simulink library "carnotUIBK"  (R2018b)
settings: Solver=VariableStepAuto  StartTime=0.0  StopTime=10.0  RelTol=1e-3  EnableMultiTasking=on
values from neighbouring files (symbols this model uses):
  A = 7*10*2    (= 140)    [theta_ground_v1.m]    (also in xlswrite1.m = num2cell(data))
  amb_factor = 1    [DOOR.m]    (also in WALL.m; WINDOW.m = 0)
  area = obj.width * obj.height    [DOOR.m]    (also in RES.m = []; ROOM.m = 0; THERMALZONE.m = area + room(kk).area; WALL.m = area - obj.doors(jj).calc_area())
  B = A/(0.5 * P)    (= 8.23529411765)    [theta_ground_v1.m]
  boundary = BOUNDARY()    [BUILDING.m]    (also in WALL.m = '')
  building = obj    [BUILDING.m]    (also in create_building_automatic.m = building.save(); ini_building_automatic.m = building.add_variant_hvac(building.variant_hvac, hvac); load_building_automatic.m = building.save())
  C = zeros(1,length(d)+1)    [CONSTRUCTION.m]    (also in DOOR.m = [0 0 0]; WALL.m = [0 0 0]; WINDOW.m = [0 0 0])
  control = 2    [GAIN.m]    (also in GAINS.m)
  cp = str2num(value)    [CONSTRUCTION.m]
  height = 0    [DOOR.m]    (also in ROOM.m; THERMALZONE.m; WALL.m; WINDOW.m)
  p = [timevec_weather weather(:,12)]    [BOUNDARY.m]    (also in WEATHER.m = 0; init_carnotUIBK.m = cell2mat(carnotUIBKpaths(i,2)))
  rho = str2num(value)    [CONSTRUCTION.m]    (also in theta_ground_v1.m = 2000)
  type = 1    [CONSTRUCTION.m]    (also in GAINS.m = raw_moisture{ii,3}; STRUCTURE.m = 0)
  view_factor = 1    [DOOR.m]    (also in WINDOW.m = 0)
  wall = []    [ROOM.m]
  z = obj.Z    [WALL.m]    (also in theta_ground_v1.m = 0)
  zone = obj.zone(ind)    [THERMALZONE.m]
undefined symbols (not defined in the file or in its folder): const, Dd, get_building, pos, Qdot_C, Qdot_H, Qdot_I_electricity, Qdot_I_light, Qdot_I_person, Qdot_S, Qdot_T_ground, Qdot_T_neighbour, Qdot_T_opaque, Qdot_T_window, Qdot_V_infiltration, Qdot_V_mech, Qdot_V_window, r_frame, solar_ratio, solar_ratio1, solar_ratio2, Tc, Tr, Ts, Uvalue, wallsurface, window, window_height, window_heigth, window_width, windowsurface, x_CO2, x_H2O, x_VOC
libraries: carnot x104, simulink x16, $bdroot x16, simulink_extras x14
(part 2 of 12)

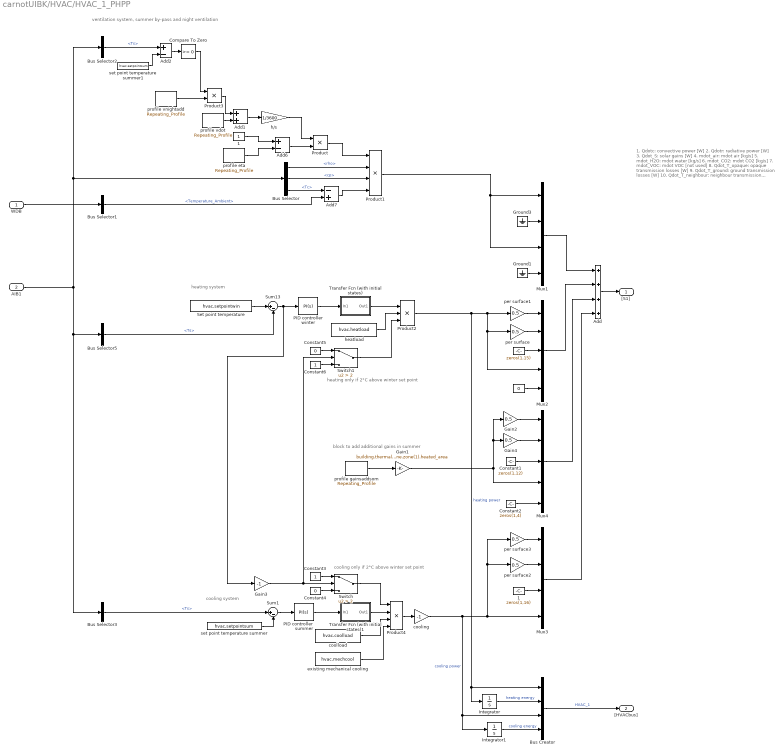
== system carnotUIBK/HVAC/HVAC_1_PHPP ==
  note: cooling only if 2°C above winter set point
  note: block to add additional gains in summer
  note: heating only if 2°C above winter set point
  note: 1.	Qdotc: convective power [W]
      | 2.	Qdotr: radiative power [W]
      | 3.	Qdot_S: solar gains [W]
      | 4.	mdot_air: mdot air [kg/s]
      | 5.	mdot_H2O: mdot water [kg/s]
      | 6.	mdot_CO2: mdot CO2 [kg/s]
      | 7.	mdot_VOC: mdot VOC [not used]
      | 8.	Qdot_T_opaque: opaque transmission losses [W]
      | 9.	Qdot_T_ground: ground transmission losses [W]
      | 10.	Qdot_T_neighbour: neighbour transmission losses [W]
      | 11.	Qdot_T_window: window transmission losses [W]
      | 12.	Qdot_V_mech: mechanical ventilation losses [W]
      | 13.	Qdot_V_window: window ventilation losses [W]
      | 14.	Qdot_V_infiltration: infiltration ventilation losses [W]
      | 15.	Qdot_I_person: person internal gains [W]
      | 16.	Qdot_I_light: light internal gains [W]
      | 17.	Qdot_I_electricity: electricity internal gains [W]
      | 18.	Qdot_H: heating power [W]
      | 19.	Qdot_C: cooling power [W]
  note: heating system
  note: cooling system
  note: ventilation system, summer by-pass and night ventilation
  WDB : Inport
  AIB1 : Inport  Port=2
  " " : Constant  Value=0
  "   " : Constant  Value=zeros(1,15)
  "   1" : Constant  Value=zeros(1,16)
  1 : Constant
  Add : Sum  Inputs=++++
  Add1 : Sum
  Add2 : Sum  Inputs=+-
  Add6 : Sum  Inputs=+-
  Add7 : Sum  Inputs=-+
  Bus Creator : BusCreator  Inputs=4
  Bus Selector : BusSelector  OutputSignals=rho,cp,Tc
  Bus Selector1 : BusSelector  OutputSignals=Temperature_Ambient
  Bus Selector2 : BusSelector  OutputSignals=Ts
  Bus Selector3 : BusSelector  OutputSignals=Ts
  Bus Selector5 : BusSelector  OutputSignals=Ts
  Compare To Zero : simulink/Logic and Bit Operations/Compare To Zero  relop=>=  OutDataTypeStr=boolean
  Constant1 : Constant  Value=zeros(1,12)
  Constant2 : Constant  Value=zeros(1,4)
  Constant3 : Constant
  Constant4 : Constant  Value=0
  Constant5 : Constant  Value=0
  Constant6 : Constant
  Gain1 : Gain  Gain=building.thermalzone.zone(1).heated_area  SaturateOnIntegerOverflow=on  OutDataTypeStr=Inherit: Same as input  ParamDataTypeStr=Inherit: Same as input
  Gain2 : Gain  Gain=0.5  SaturateOnIntegerOverflow=on  OutDataTypeStr=Inherit: Same as input  ParamDataTypeStr=Inherit: Same as input
  Gain3 : Gain  Gain=-1  SaturateOnIntegerOverflow=on  OutDataTypeStr=Inherit: Same as input  ParamDataTypeStr=Inherit: Same as input
  Gain4 : Gain  Gain=0.5  SaturateOnIntegerOverflow=on  OutDataTypeStr=Inherit: Same as input  ParamDataTypeStr=Inherit: Same as input
  Ground1 : Ground
  Ground3 : Ground
  Integrator : Integrator
  Integrator1 : Integrator
  Mux1 : Mux  Inputs=[1 10 1 7]
  Mux2 : Mux  Inputs=[1 1 15 1 1]
  Mux3 : Mux  Inputs=[1 1 16 1]
  Mux4 : Mux  Inputs=[1 1 12 1 4]
  PID controller summer : simulink/Continuous/PID Controller  Controller=PI  Form=Ideal  TimeDomain=Continuous-time  SampleTime=-1  IntegratorMethod=Forward Euler  FilterMethod=Forward Euler  ControllerParametersSource=internal  P=hvac.valves.Kp  I=(1/(hvac.valves.Tn*60))  D=0  UseFilter=on  N=100  TunerSelectOption=Transfer Function Based (PID Tuner App)  InitialConditionSource=internal  InitialConditionForIntegrator=0  InitialConditionForFilter=0  DifferentiatorICPrevScaledInput=0  ExternalReset=none  TrackingMode=off  Kt=1  LimitOutput=on  UpperSaturationLimit=hvac.valves.valve_up  LowerSaturationLimit=hvac.valves.valve_low  LinearizeAsGain=off  AntiWindupMode=clamping  Kb=1  POutMin=[]  POutMax=[]  IOutMin=[]  IOutMax=[]  DOutMin=[]  DOutMax=[]  NOutMin=[]  NOutMax=[]  SumOutMin=[]  SumOutMax=[]  SaturationOutMin=[]  SaturationOutMax=[]  PParamMin=[]  PParamMax=[]  IParamMin=[]  IParamMax=[]  DParamMin=[]  DParamMax=[]  NParamMin=[]  NParamMax=[]  KbParamMin=[]  KbParamMax=[]  KtParamMin=[]  KtParamMax=[]  KbOutMin=[]  KbOutMax=[]  KtOutMin=[]  KtOutMax=[]  IntegratorOutMin=[]  IntegratorOutMax=[]  FilterOutMin=[]  FilterOutMax=[]  SumI1OutMin=[]  SumI1OutMax=[]  SumI2OutMin=[]  SumI2OutMax=[]  SumI3OutMin=[]  SumI3OutMax=[]  SumI4OutMin=[]  SumI4OutMax=[]  SumDOutMin=[]  SumDOutMax=[]  DifferentiatorOutMin=[]  DifferentiatorOutMax=[]  FilterDiffOutCoefMin=[]  FilterDiffOutCoefMax=[]  ReciprocalOutMin=[]  ReciprocalOutMax=[]  SumDenOutMin=[]  SumDenOutMax=[]  SumNumOutMin=[]  SumNumOutMax=[]  DivideOutMin=[]  DivideOutMax=[]  IntegratorContinuousStateAttributes=''  IntegratorStateMustResolveToSignalObject=off  IntegratorRTWStateStorageClass=Auto  FilterContinuousStateAttributes=''  FilterStateMustResolveToSignalObject=off  FilterRTWStateStorageClass=Auto  ParallelPVariant=Passthrough  IdealPVariant=InternalParameters  IVariant=InternalParameters  DVariant=Disabled  IntegratorVariant=Continuous  SatVariant=Enabled  AWVariant=ContClampingIdeal  PCopyVariant=InternalParamsIdeal  TRVariant=Disabled  FdbkBlocksVariant=Forward  IdealPFdbkVariant=Disabled  SatFdbkVariant=Disabled  DerivativeFilterVariant=Disabled  NVariant=Disabled  NCopyVariant=Disabled_SignalSpec  FilterICVariant=Disabled  IntegratorICVariant=InternalICs  ExternalResetVariant=Disabled  TRSumVariant=Passthrough  SumFdbkVariant=Disabled  SumVariant=Sum_PI
  PID controller winter : simulink/Continuous/PID Controller  Controller=PI  Form=Ideal  TimeDomain=Continuous-time  SampleTime=-1  IntegratorMethod=Forward Euler  FilterMethod=Forward Euler  ControllerParametersSource=internal  P=hvac.valves.Kp  I=(1/(hvac.valves.Tn*60))  D=0  UseFilter=on  N=100  TunerSelectOption=Transfer Function Based (PID Tuner App)  InitialConditionSource=internal  InitialConditionForIntegrator=0  InitialConditionForFilter=0  DifferentiatorICPrevScaledInput=0  ExternalReset=none  TrackingMode=off  Kt=1  LimitOutput=on  UpperSaturationLimit=hvac.valves.valve_up  LowerSaturationLimit=hvac.valves.valve_low  LinearizeAsGain=off  AntiWindupMode=clamping  Kb=1  POutMin=[]  POutMax=[]  IOutMin=[]  IOutMax=[]  DOutMin=[]  DOutMax=[]  NOutMin=[]  NOutMax=[]  SumOutMin=[]  SumOutMax=[]  SaturationOutMin=[]  SaturationOutMax=[]  PParamMin=[]  PParamMax=[]  IParamMin=[]  IParamMax=[]  DParamMin=[]  DParamMax=[]  NParamMin=[]  NParamMax=[]  KbParamMin=[]  KbParamMax=[]  KtParamMin=[]  KtParamMax=[]  KbOutMin=[]  KbOutMax=[]  KtOutMin=[]  KtOutMax=[]  IntegratorOutMin=[]  IntegratorOutMax=[]  FilterOutMin=[]  FilterOutMax=[]  SumI1OutMin=[]  SumI1OutMax=[]  SumI2OutMin=[]  SumI2OutMax=[]  SumI3OutMin=[]  SumI3OutMax=[]  SumI4OutMin=[]  SumI4OutMax=[]  SumDOutMin=[]  SumDOutMax=[]  DifferentiatorOutMin=[]  DifferentiatorOutMax=[]  FilterDiffOutCoefMin=[]  FilterDiffOutCoefMax=[]  ReciprocalOutMin=[]  ReciprocalOutMax=[]  SumDenOutMin=[]  SumDenOutMax=[]  SumNumOutMin=[]  SumNumOutMax=[]  DivideOutMin=[]  DivideOutMax=[]  IntegratorContinuousStateAttributes=''  IntegratorStateMustResolveToSignalObject=off  IntegratorRTWStateStorageClass=Auto  FilterContinuousStateAttributes=''  FilterStateMustResolveToSignalObject=off  FilterRTWStateStorageClass=Auto  ParallelPVariant=Passthrough  IdealPVariant=InternalParameters  IVariant=InternalParameters  DVariant=Disabled  IntegratorVariant=Continuous  SatVariant=Enabled  AWVariant=ContClampingIdeal  PCopyVariant=InternalParamsIdeal  TRVariant=Disabled  FdbkBlocksVariant=Forward  IdealPFdbkVariant=Disabled  SatFdbkVariant=Disabled  DerivativeFilterVariant=Disabled  NVariant=Disabled  NCopyVariant=Disabled_SignalSpec  FilterICVariant=Disabled  IntegratorICVariant=InternalICs  ExternalResetVariant=Disabled  TRSumVariant=Passthrough  SumFdbkVariant=Disabled  SumVariant=Sum_PI
  Product : Product
  Product1 : Product  Inputs=4
  Product2 : Product  Inputs=3
  Product3 : Product
  Product4 : Product  Inputs=4
  Set point temperature : Constant  Value=hvac.setpointwin  VectorParams1D=off
  Sum1 : Sum  Inputs=|+-
  Sum13 : Sum  Inputs=|+-
  Switch : Switch  Criteria=u2 > Threshold  Threshold=2
  Switch1 : Switch  Criteria=u2 > Threshold  Threshold=2
  Transfer Fcn (with initial states) : Subsystem  mask(Transfer Function with Initial States){N=[1], D=[300  1], X0=0}
      mask prompts: N "Numerator:"; D "Denominator:"; X0 "Initial conditions:"
      mask help: Vector expressions for numerator, and denominator. Coefficients are in descending powers of s.
      mask init:
      | [A,B,C,Dd]=tf2ss(N,D);if (isempty(X0));[m,n]=size(A);X0=zeros(1,m); end;
      mask Help: Specify the initial states for the transfer function.  The state ordering is determined by the m-file tf2ss.  There is no unique mapping of the states in a transfer function to states in a state-space representation.  However, tf2ss will consistently use the same mapping for a given transfer function.
      mask Display: dpoly(N,D,'s')
  Transfer Fcn (with initial states)1 : Subsystem  mask(Transfer Function with Initial States){N=[1], D=[300  1], X0=0}
      mask prompts: N "Numerator:"; D "Denominator:"; X0 "Initial conditions:"
      mask help: Vector expressions for numerator, and denominator. Coefficients are in descending powers of s.
      mask init:
      | [A,B,C,Dd]=tf2ss(N,D);if (isempty(X0));[m,n]=size(A);X0=zeros(1,m); end;
      mask Help: Specify the initial states for the transfer function.  The state ordering is determined by the m-file tf2ss.  There is no unique mapping of the states in a transfer function to states in a state-space representation.  However, tf2ss will consistently use the same mapping for a given transfer function.
      mask Display: dpoly(N,D,'s')
  cooling : Gain  Gain=-1  SaturateOnIntegerOverflow=on  OutDataTypeStr=Inherit: Same as input  ParamDataTypeStr=Inherit: Same as input
  coolload : Constant  Value=hvac.coolload
  existing mechanical cooling : Constant  Value=hvac.mechcool
  h/s : Gain  Gain=1/3600
  heatload : Constant  Value=hvac.heatload
  per surface{,1..3} (4 alike) : Gain  Gain=0.5  SaturateOnIntegerOverflow=on  OutDataTypeStr=Inherit: Same as input  ParamDataTypeStr=Inherit: Same as input
  profile eta : carnot/Load/General/Repeating_Profile  period=hvac.eta.time(end)  rep_seq_t=hvac.eta.time(1:end-1)  rep_seq_d=hvac.eta.duration  rep_seq_y=hvac.eta.value
  profile gainsaddsom : carnot/Load/General/Repeating_Profile  period=hvac.gainsum.time(end)  rep_seq_t=hvac.gainsum.time(1:end-1)  rep_seq_d=hvac.gainsum.duration  rep_seq_y=hvac.gainsum.value
  profile vdot : carnot/Load/General/Repeating_Profile  period=hvac.vdot_winsom.time(end)  rep_seq_t=hvac.vdot_winsom.time(1:end-1)  rep_seq_d=hvac.vdot_winsom.duration  rep_seq_y=hvac.vdot_winsom.value
  profile vnightadd : carnot/Load/General/Repeating_Profile  period=hvac.night_vent_s.time(end)  rep_seq_t=hvac.night_vent_s.time(1:end-1)  rep_seq_d=hvac.night_vent_s.duration  rep_seq_y=hvac.night_vent_s.value
  set point temperature summer : Constant  Value=hvac.setpointsum  VectorParams1D=off
  set point temperature summer1 : Constant  Value=hvac.setpointsum  VectorParams1D=off
  "[S1]" : Outport  InitialOutput=0
  "[HVACbus]" : Outport  Port=2  InitialOutput=0
  wires:
  profile eta/1 -> Add6/2
  profile vdot/1 -> Add1/2
  1/1 -> Add6/1
  Add6/1 -> Product/2
  Product/1 -> Product1/1
  Bus Selector/1 -> Product1/2  "<rho>"
  Bus Selector/2 -> Product1/3  "<cp>"
  Bus Selector/3 -> Add7/1  "<Tc>"
  Product1/1 -> Mux1/3, Mux1/1
  Ground3/1 -> Mux1/2
  WDB/1 -> Bus Selector1/1
  Bus Selector1/1 -> Add7/2  "<Temperature_Ambient>"
  Add7/1 -> Product1/4
  Ground1/1 -> Mux1/4
  h/s/1 -> Product/1
  Add/1 -> "[S1]"/1
  Mux2/1 -> Add/2
  Mux1/1 -> Add/1
  Sum13/1 -> PID controller winter/1, Gain3/1
  Set point temperature/1 -> Sum13/1
  Bus Selector5/1 -> Sum13/2  "<Ts>"
  PID controller winter/1 -> Transfer Fcn (with initial states)/1(In1)
  heatload/1 -> Product2/2
  per surface/1 -> Mux2/2
  per surface1/1 -> Mux2/1
  Transfer Fcn (with initial states)/1(Out1) -> Product2/1
  " "/1 -> Mux2/5
  "   "/1 -> Mux2/3
  Add1/1 -> h/s/1
  Product3/1 -> Add1/1
  profile vnightadd/1 -> Product3/2
  Bus Selector2/1 -> Add2/1  "<Ts>"
  set point temperature summer1/1 -> Add2/2
  Add2/1 -> Compare To Zero/1
  Compare To Zero/1 -> Product3/1
  Constant2/1 -> Mux4/5
  Constant1/1 -> Mux4/3
  profile gainsaddsom/1 -> Gain1/1
  Gain2/1 -> Mux4/1
  Gain4/1 -> Mux4/2
  Gain1/1 -> Mux4/4, Gain2/1, Gain4/1
  Mux4/1 -> Add/3
  Mux3/1 -> Add/4
  Sum1/1 -> PID controller summer/1
  set point temperature summer/1 -> Sum1/2
  Bus Selector3/1 -> Sum1/1  "<Ts>"
  PID controller summer/1 -> Transfer Fcn (with initial states)1/1(In1)
  coolload/1 -> Product4/3
  Product4/1 -> cooling/1
  per surface2/1 -> Mux3/2
  per surface3/1 -> Mux3/1
  Transfer Fcn (with initial states)1/1(Out1) -> Product4/2
  AIB1/1 -> Bus Selector3/1, Bus Selector5/1, Bus Selector/1, Bus Selector2/1
  "   1"/1 -> Mux3/3
  existing mechanical cooling/1 -> Product4/4
  Constant3/1 -> Switch/1
  Constant4/1 -> Switch/3
  Switch/1 -> Product4/1
  Gain3/1 -> Switch1/2, Switch/2
  Constant5/1 -> Switch1/1
  Constant6/1 -> Switch1/3
  Switch1/1 -> Product2/3
  Bus Creator/1 -> "[HVACbus]"/1  "HVAC_1"
  Integrator/1 -> Bus Creator/2  "heating energy"
  Product2/1 -> per surface1/1, Mux2/4, per surface/1, Integrator/1, Bus Creator/1  "heating power"
  Integrator1/1 -> Bus Creator/4  "cooling energy"
  cooling/1 -> Bus Creator/3, Integrator1/1, per surface3/1, per surface2/1, Mux3/4  "cooling power"

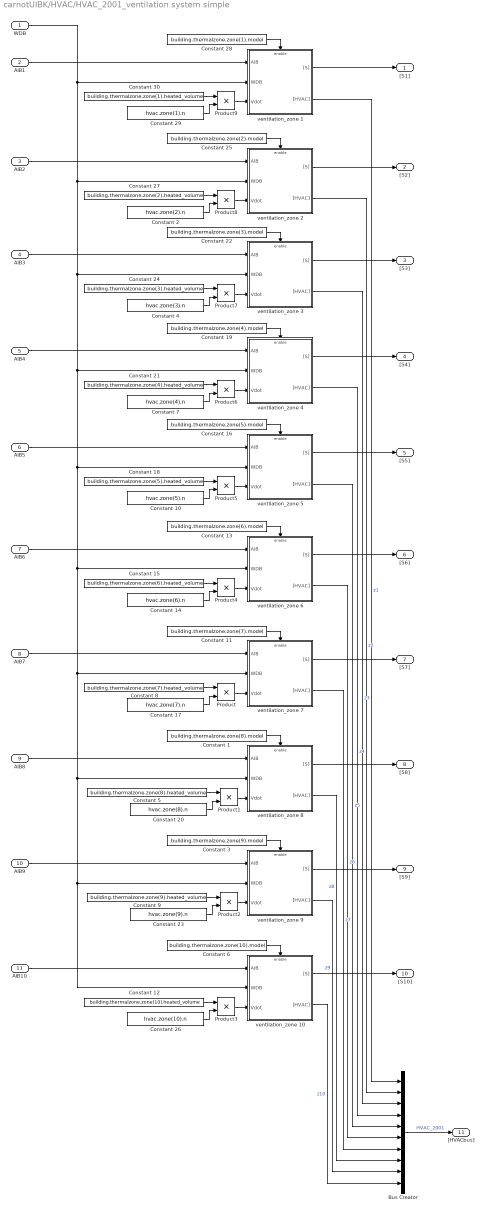
== system carnotUIBK/HVAC/HVAC_2001_ventilation system simple ==
  WDB : Inport
  AIB1 : Inport  Port=2
  AIB2 : Inport  Port=3
  AIB3 : Inport  Port=4
  AIB4 : Inport  Port=5
  AIB5 : Inport  Port=6
  AIB6 : Inport  Port=7
  AIB7 : Inport  Port=8
  "AIB8 " : Inport  Port=9
  AIB9 : Inport  Port=10
  AIB10 : Inport  Port=11
  Bus Creator : BusCreator  Inputs=10
  Constant 1 : Constant  Value=building.thermalzone.zone(8).model  VectorParams1D=off
  Constant 10 : Constant  Value=hvac.zone(5).n  VectorParams1D=off
  Constant 11 : Constant  Value=building.thermalzone.zone(7).model  VectorParams1D=off
  Constant 12 : Constant  Value=building.thermalzone.zone(10).heated_volume  VectorParams1D=off
  Constant 13 : Constant  Value=building.thermalzone.zone(6).model  VectorParams1D=off
  Constant 14 : Constant  Value=hvac.zone(6).n  VectorParams1D=off
  Constant 15 : Constant  Value=building.thermalzone.zone(6).heated_volume  VectorParams1D=off
  Constant 16 : Constant  Value=building.thermalzone.zone(5).model  VectorParams1D=off
  Constant 17 : Constant  Value=hvac.zone(7).n  VectorParams1D=off
  Constant 18 : Constant  Value=building.thermalzone.zone(5).heated_volume  VectorParams1D=off
  Constant 19 : Constant  Value=building.thermalzone.zone(4).model  VectorParams1D=off
  Constant 2 : Constant  Value=hvac.zone(2).n  VectorParams1D=off
  Constant 20 : Constant  Value=hvac.zone(8).n  VectorParams1D=off
  Constant 21 : Constant  Value=building.thermalzone.zone(4).heated_volume  VectorParams1D=off
  Constant 22 : Constant  Value=building.thermalzone.zone(3).model  VectorParams1D=off
  Constant 23 : Constant  Value=hvac.zone(9).n  VectorParams1D=off
  Constant 24 : Constant  Value=building.thermalzone.zone(3).heated_volume  VectorParams1D=off
  Constant 25 : Constant  Value=building.thermalzone.zone(2).model  VectorParams1D=off
  Constant 26 : Constant  Value=hvac.zone(10).n  VectorParams1D=off
  Constant 27 : Constant  Value=building.thermalzone.zone(2).heated_volume  VectorParams1D=off
  Constant 28 : Constant  Value=building.thermalzone.zone(1).model  VectorParams1D=off
  Constant 29 : Constant  Value=hvac.zone(1).n  VectorParams1D=off
  Constant 3 : Constant  Value=building.thermalzone.zone(9).model  VectorParams1D=off
  Constant 30 : Constant  Value=building.thermalzone.zone(1).heated_volume  VectorParams1D=off
  Constant 4 : Constant  Value=hvac.zone(3).n  VectorParams1D=off
  Constant 5 : Constant  Value=building.thermalzone.zone(8).heated_volume  VectorParams1D=off
  Constant 6 : Constant  Value=building.thermalzone.zone(10).model  VectorParams1D=off
  Constant 7 : Constant  Value=hvac.zone(4).n  VectorParams1D=off
  Constant 8 : Constant  Value=building.thermalzone.zone(7).heated_volume  VectorParams1D=off
  Constant 9 : Constant  Value=building.thermalzone.zone(9).heated_volume  VectorParams1D=off
  Product{,1..9} (10 alike) : Product
  ventilation_zone 1 : Subsystem  mask(ACTIVE COMPONENT){co2=400, eta=hvac.zone(1).eta, eta_x=hvac.zone(1).eta_x}
      mask prompts: co2 "CO2 content of air in ppm"; eta "heat recovery efficiency"; eta_x "moisture recovery efficiency"
      mask help:
      | This block represents the AIR VENTILATION from outdoors into a zone.
      |
      | r : rate of nominal air flow between outdoors and indoor, [0,1]
      | [S] : vector for sinks and sources.
      |
      | NOTE: Mass flows of water and CO2 are taken into consideration.
      |
      | ASSUMPTION:
      | Incoming air volume flow is identical to outgoing air volume flow.
      mask init:
      | CO2norm = co2*1e-6;
      mask Help: web(fullfile(path_carnot('help'),'Ventilation_AIV.html'),'-helpbrowser')
      mask Display:
      | plot([0.2 0.35], [0.8 0.7])
      | plot([0.35 0.65], [0.7 0.7])
      | plot([0.65 0.8], [0.7 0.8])
      | plot([0.65 0.8], [0.76 0.8])
      | plot([0.7 0.8], [0.65 0.8])
      | 
      | plot([0.2 0.35], [0.2 0.3])
      | plot([0.35 0.65], [0.3 0.3])
      | plot([0.65 0.8], [0.3 0.2])
      | plot([0.2 0.25], [0.2 0.32])
      | plot([0.2 0.35], [0.2 0.23])
      | 
      | plot ([0.45 0.45], [0 1])
      | plot ([0.55 0.55], [0 1])
      | 
      | plot ([0.45 0.55], [0.2 0.2])
      | plot ([0.45 0.55], [0.8 0.8])
      | 
      | plot ([0.45 0.55], [0 0.2])
      | plot ([0.45 0.55], [0.8 1])
  ventilation_zone 10 : Subsystem  mask(ACTIVE COMPONENT){co2=400, eta=hvac.zone(10).eta, eta_x=hvac.zone(10).eta_x}
      mask prompts: co2 "CO2 content of air in ppm"; eta "heat recovery efficiency"; eta_x "moisture recovery efficiency"
      mask help:
      | This block represents the AIR VENTILATION from outdoors into a zone.
      |
      | r : rate of nominal air flow between outdoors and indoor, [0,1]
      | [S] : vector for sinks and sources.
      |
      | NOTE: Mass flows of water and CO2 are taken into consideration.
      |
      | ASSUMPTION:
      | Incoming air volume flow is identical to outgoing air volume flow.
      mask init:
      | CO2norm = co2*1e-6;
      mask Help: web(fullfile(path_carnot('help'),'Ventilation_AIV.html'),'-helpbrowser')
      mask Display:
      | plot([0.2 0.35], [0.8 0.7])
      | plot([0.35 0.65], [0.7 0.7])
      | plot([0.65 0.8], [0.7 0.8])
      | plot([0.65 0.8], [0.76 0.8])
      | plot([0.7 0.8], [0.65 0.8])
      | 
      | plot([0.2 0.35], [0.2 0.3])
      | plot([0.35 0.65], [0.3 0.3])
      | plot([0.65 0.8], [0.3 0.2])
      | plot([0.2 0.25], [0.2 0.32])
      | plot([0.2 0.35], [0.2 0.23])
      | 
      | plot ([0.45 0.45], [0 1])
      | plot ([0.55 0.55], [0 1])
      | 
      | plot ([0.45 0.55], [0.2 0.2])
      | plot ([0.45 0.55], [0.8 0.8])
      | 
      | plot ([0.45 0.55], [0 0.2])
      | plot ([0.45 0.55], [0.8 1])
  ventilation_zone 2 : Subsystem  mask(ACTIVE COMPONENT){co2=400, eta=hvac.zone(2).eta, eta_x=hvac.zone(2).eta_x}
      mask prompts: co2 "CO2 content of air in ppm"; eta "heat recovery efficiency"; eta_x "moisture recovery efficiency"
      mask help:
      | This block represents the AIR VENTILATION from outdoors into a zone.
      |
      | r : rate of nominal air flow between outdoors and indoor, [0,1]
      | [S] : vector for sinks and sources.
      |
      | NOTE: Mass flows of water and CO2 are taken into consideration.
      |
      | ASSUMPTION:
      | Incoming air volume flow is identical to outgoing air volume flow.
      mask init:
      | CO2norm = co2*1e-6;
      mask Help: web(fullfile(path_carnot('help'),'Ventilation_AIV.html'),'-helpbrowser')
      mask Display:
      | plot([0.2 0.35], [0.8 0.7])
      | plot([0.35 0.65], [0.7 0.7])
      | plot([0.65 0.8], [0.7 0.8])
      | plot([0.65 0.8], [0.76 0.8])
      | plot([0.7 0.8], [0.65 0.8])
      | 
      | plot([0.2 0.35], [0.2 0.3])
      | plot([0.35 0.65], [0.3 0.3])
      | plot([0.65 0.8], [0.3 0.2])
      | plot([0.2 0.25], [0.2 0.32])
      | plot([0.2 0.35], [0.2 0.23])
      | 
      | plot ([0.45 0.45], [0 1])
      | plot ([0.55 0.55], [0 1])
      | 
      | plot ([0.45 0.55], [0.2 0.2])
      | plot ([0.45 0.55], [0.8 0.8])
      | 
      | plot ([0.45 0.55], [0 0.2])
      | plot ([0.45 0.55], [0.8 1])
  ventilation_zone 3 : Subsystem  mask(ACTIVE COMPONENT){co2=400, eta=hvac.zone(3).eta, eta_x=hvac.zone(3).eta_x}
      mask prompts: co2 "CO2 content of air in ppm"; eta "heat recovery efficiency"; eta_x "moisture recovery efficiency"
      mask help:
      | This block represents the AIR VENTILATION from outdoors into a zone.
      |
      | r : rate of nominal air flow between outdoors and indoor, [0,1]
      | [S] : vector for sinks and sources.
      |
      | NOTE: Mass flows of water and CO2 are taken into consideration.
      |
      | ASSUMPTION:
      | Incoming air volume flow is identical to outgoing air volume flow.
      mask init:
      | CO2norm = co2*1e-6;
      mask Help: web(fullfile(path_carnot('help'),'Ventilation_AIV.html'),'-helpbrowser')
      mask Display:
      | plot([0.2 0.35], [0.8 0.7])
      | plot([0.35 0.65], [0.7 0.7])
      | plot([0.65 0.8], [0.7 0.8])
      | plot([0.65 0.8], [0.76 0.8])
      | plot([0.7 0.8], [0.65 0.8])
      | 
      | plot([0.2 0.35], [0.2 0.3])
      | plot([0.35 0.65], [0.3 0.3])
      | plot([0.65 0.8], [0.3 0.2])
      | plot([0.2 0.25], [0.2 0.32])
      | plot([0.2 0.35], [0.2 0.23])
      | 
      | plot ([0.45 0.45], [0 1])
      | plot ([0.55 0.55], [0 1])
      | 
      | plot ([0.45 0.55], [0.2 0.2])
      | plot ([0.45 0.55], [0.8 0.8])
      | 
      | plot ([0.45 0.55], [0 0.2])
      | plot ([0.45 0.55], [0.8 1])
  ventilation_zone 4 : Subsystem  mask(ACTIVE COMPONENT){co2=400, eta=hvac.zone(4).eta, eta_x=hvac.zone(4).eta_x}
      mask prompts: co2 "CO2 content of air in ppm"; eta "heat recovery efficiency"; eta_x "moisture recovery efficiency"
      mask help:
      | This block represents the AIR VENTILATION from outdoors into a zone.
      |
      | r : rate of nominal air flow between outdoors and indoor, [0,1]
      | [S] : vector for sinks and sources.
      |
      | NOTE: Mass flows of water and CO2 are taken into consideration.
      |
      | ASSUMPTION:
      | Incoming air volume flow is identical to outgoing air volume flow.
      mask init:
      | CO2norm = co2*1e-6;
      mask Help: web(fullfile(path_carnot('help'),'Ventilation_AIV.html'),'-helpbrowser')
      mask Display:
      | plot([0.2 0.35], [0.8 0.7])
      | plot([0.35 0.65], [0.7 0.7])
      | plot([0.65 0.8], [0.7 0.8])
      | plot([0.65 0.8], [0.76 0.8])
      | plot([0.7 0.8], [0.65 0.8])
      | 
      | plot([0.2 0.35], [0.2 0.3])
      | plot([0.35 0.65], [0.3 0.3])
      | plot([0.65 0.8], [0.3 0.2])
      | plot([0.2 0.25], [0.2 0.32])
      | plot([0.2 0.35], [0.2 0.23])
      | 
      | plot ([0.45 0.45], [0 1])
      | plot ([0.55 0.55], [0 1])
      | 
      | plot ([0.45 0.55], [0.2 0.2])
      | plot ([0.45 0.55], [0.8 0.8])
      | 
      | plot ([0.45 0.55], [0 0.2])
      | plot ([0.45 0.55], [0.8 1])
  ventilation_zone 5 : Subsystem  mask(ACTIVE COMPONENT){co2=400, eta=hvac.zone(5).eta, eta_x=hvac.zone(5).eta_x}
      mask prompts: co2 "CO2 content of air in ppm"; eta "heat recovery efficiency"; eta_x "moisture recovery efficiency"
      mask help:
      | This block represents the AIR VENTILATION from outdoors into a zone.
      |
      | r : rate of nominal air flow between outdoors and indoor, [0,1]
      | [S] : vector for sinks and sources.
      |
      | NOTE: Mass flows of water and CO2 are taken into consideration.
      |
      | ASSUMPTION:
      | Incoming air volume flow is identical to outgoing air volume flow.
      mask init:
      | CO2norm = co2*1e-6;
      mask Help: web(fullfile(path_carnot('help'),'Ventilation_AIV.html'),'-helpbrowser')
      mask Display:
      | plot([0.2 0.35], [0.8 0.7])
      | plot([0.35 0.65], [0.7 0.7])
      | plot([0.65 0.8], [0.7 0.8])
      | plot([0.65 0.8], [0.76 0.8])
      | plot([0.7 0.8], [0.65 0.8])
      | 
      | plot([0.2 0.35], [0.2 0.3])
      | plot([0.35 0.65], [0.3 0.3])
      | plot([0.65 0.8], [0.3 0.2])
      | plot([0.2 0.25], [0.2 0.32])
      | plot([0.2 0.35], [0.2 0.23])
      | 
      | plot ([0.45 0.45], [0 1])
      | plot ([0.55 0.55], [0 1])
      | 
      | plot ([0.45 0.55], [0.2 0.2])
      | plot ([0.45 0.55], [0.8 0.8])
      | 
      | plot ([0.45 0.55], [0 0.2])
      | plot ([0.45 0.55], [0.8 1])
  ventilation_zone 6 : Subsystem  mask(ACTIVE COMPONENT){co2=400, eta=hvac.zone(6).eta, eta_x=hvac.zone(6).eta_x}
      mask prompts: co2 "CO2 content of air in ppm"; eta "heat recovery efficiency"; eta_x "moisture recovery efficiency"
      mask help:
      | This block represents the AIR VENTILATION from outdoors into a zone.
      |
      | r : rate of nominal air flow between outdoors and indoor, [0,1]
      | [S] : vector for sinks and sources.
      |
      | NOTE: Mass flows of water and CO2 are taken into consideration.
      |
      | ASSUMPTION:
      | Incoming air volume flow is identical to outgoing air volume flow.
      mask init:
      | CO2norm = co2*1e-6;
      mask Help: web(fullfile(path_carnot('help'),'Ventilation_AIV.html'),'-helpbrowser')
      mask Display:
      | plot([0.2 0.35], [0.8 0.7])
      | plot([0.35 0.65], [0.7 0.7])
      | plot([0.65 0.8], [0.7 0.8])
      | plot([0.65 0.8], [0.76 0.8])
      | plot([0.7 0.8], [0.65 0.8])
      | 
      | plot([0.2 0.35], [0.2 0.3])
      | plot([0.35 0.65], [0.3 0.3])
      | plot([0.65 0.8], [0.3 0.2])
      | plot([0.2 0.25], [0.2 0.32])
      | plot([0.2 0.35], [0.2 0.23])
      | 
      | plot ([0.45 0.45], [0 1])
      | plot ([0.55 0.55], [0 1])
      | 
      | plot ([0.45 0.55], [0.2 0.2])
      | plot ([0.45 0.55], [0.8 0.8])
      | 
      | plot ([0.45 0.55], [0 0.2])
      | plot ([0.45 0.55], [0.8 1])
  ventilation_zone 7 : Subsystem  mask(ACTIVE COMPONENT){co2=400, eta=hvac.zone(7).eta, eta_x=hvac.zone(7).eta_x}
      mask prompts: co2 "CO2 content of air in ppm"; eta "heat recovery efficiency"; eta_x "moisture recovery efficiency"
      mask help:
      | This block represents the AIR VENTILATION from outdoors into a zone.
      |
      | r : rate of nominal air flow between outdoors and indoor, [0,1]
      | [S] : vector for sinks and sources.
      |
      | NOTE: Mass flows of water and CO2 are taken into consideration.
      |
      | ASSUMPTION:
      | Incoming air volume flow is identical to outgoing air volume flow.
      mask init:
      | CO2norm = co2*1e-6;
      mask Help: web(fullfile(path_carnot('help'),'Ventilation_AIV.html'),'-helpbrowser')
      mask Display:
      | plot([0.2 0.35], [0.8 0.7])
      | plot([0.35 0.65], [0.7 0.7])
      | plot([0.65 0.8], [0.7 0.8])
      | plot([0.65 0.8], [0.76 0.8])
      | plot([0.7 0.8], [0.65 0.8])
      | 
      | plot([0.2 0.35], [0.2 0.3])
      | plot([0.35 0.65], [0.3 0.3])
      | plot([0.65 0.8], [0.3 0.2])
      | plot([0.2 0.25], [0.2 0.32])
      | plot([0.2 0.35], [0.2 0.23])
      | 
      | plot ([0.45 0.45], [0 1])
      | plot ([0.55 0.55], [0 1])
      | 
      | plot ([0.45 0.55], [0.2 0.2])
      | plot ([0.45 0.55], [0.8 0.8])
      | 
      | plot ([0.45 0.55], [0 0.2])
      | plot ([0.45 0.55], [0.8 1])
  ventilation_zone 8 : Subsystem  mask(ACTIVE COMPONENT){co2=400, eta=hvac.zone(8).eta, eta_x=hvac.zone(8).eta_x}
      mask prompts: co2 "CO2 content of air in ppm"; eta "heat recovery efficiency"; eta_x "moisture recovery efficiency"
      mask help:
      | This block represents the AIR VENTILATION from outdoors into a zone.
      |
      | r : rate of nominal air flow between outdoors and indoor, [0,1]
      | [S] : vector for sinks and sources.
      |
      | NOTE: Mass flows of water and CO2 are taken into consideration.
      |
      | ASSUMPTION:
      | Incoming air volume flow is identical to outgoing air volume flow.
      mask init:
      | CO2norm = co2*1e-6;
      mask Help: web(fullfile(path_carnot('help'),'Ventilation_AIV.html'),'-helpbrowser')
      mask Display:
      | plot([0.2 0.35], [0.8 0.7])
      | plot([0.35 0.65], [0.7 0.7])
      | plot([0.65 0.8], [0.7 0.8])
      | plot([0.65 0.8], [0.76 0.8])
      | plot([0.7 0.8], [0.65 0.8])
      | 
      | plot([0.2 0.35], [0.2 0.3])
      | plot([0.35 0.65], [0.3 0.3])
      | plot([0.65 0.8], [0.3 0.2])
      | plot([0.2 0.25], [0.2 0.32])
      | plot([0.2 0.35], [0.2 0.23])
      | 
      | plot ([0.45 0.45], [0 1])
      | plot ([0.55 0.55], [0 1])
      | 
      | plot ([0.45 0.55], [0.2 0.2])
      | plot ([0.45 0.55], [0.8 0.8])
      | 
      | plot ([0.45 0.55], [0 0.2])
      | plot ([0.45 0.55], [0.8 1])
  ventilation_zone 9 : Subsystem  mask(ACTIVE COMPONENT){co2=400, eta=hvac.zone(9).eta, eta_x=hvac.zone(9).eta_x}
      mask prompts: co2 "CO2 content of air in ppm"; eta "heat recovery efficiency"; eta_x "moisture recovery efficiency"
      mask help:
      | This block represents the AIR VENTILATION from outdoors into a zone.
      |
      | r : rate of nominal air flow between outdoors and indoor, [0,1]
      | [S] : vector for sinks and sources.
      |
      | NOTE: Mass flows of water and CO2 are taken into consideration.
      |
      | ASSUMPTION:
      | Incoming air volume flow is identical to outgoing air volume flow.
      mask init:
      | CO2norm = co2*1e-6;
      mask Help: web(fullfile(path_carnot('help'),'Ventilation_AIV.html'),'-helpbrowser')
      mask Display:
      | plot([0.2 0.35], [0.8 0.7])
      | plot([0.35 0.65], [0.7 0.7])
      | plot([0.65 0.8], [0.7 0.8])
      | plot([0.65 0.8], [0.76 0.8])
      | plot([0.7 0.8], [0.65 0.8])
      | 
      | plot([0.2 0.35], [0.2 0.3])
      | plot([0.35 0.65], [0.3 0.3])
      | plot([0.65 0.8], [0.3 0.2])
      | plot([0.2 0.25], [0.2 0.32])
      | plot([0.2 0.35], [0.2 0.23])
      | 
      | plot ([0.45 0.45], [0 1])
      | plot ([0.55 0.55], [0 1])
      | 
      | plot ([0.45 0.55], [0.2 0.2])
      | plot ([0.45 0.55], [0.8 0.8])
      | 
      | plot ([0.45 0.55], [0 0.2])
      | plot ([0.45 0.55], [0.8 1])
  "[S1]" : Outport
  "[S2]" : Outport  Port=2
  "[S3]" : Outport  Port=3
  "[S4]" : Outport  Port=4
  "[S5]" : Outport  Port=5
  "[S6]" : Outport  Port=6
  "[S7]" : Outport  Port=7
  "[S8]" : Outport  Port=8
  "[S9]" : Outport  Port=9
  "[S10]" : Outport  Port=10
  "[HVACbus]" : Outport  Port=11  InitialOutput=0
  wires:
  AIB7/1 -> ventilation_zone 7/1(AIB)
  ventilation_zone 7/1("[S]") -> "[S7]"/1
  Constant 11/1 -> ventilation_zone 7/Enable
  "AIB8 "/1 -> ventilation_zone 8/1(AIB)
  Product1/1 -> ventilation_zone 8/3(Vdot)
  ventilation_zone 8/1("[S]") -> "[S8]"/1
  Constant 1/1 -> ventilation_zone 8/Enable
  AIB9/1 -> ventilation_zone 9/1(AIB)
  Product2/1 -> ventilation_zone 9/3(Vdot)
  ventilation_zone 9/1("[S]") -> "[S9]"/1
  Constant 3/1 -> ventilation_zone 9/Enable
  AIB10/1 -> ventilation_zone 10/1(AIB)
  Product3/1 -> ventilation_zone 10/3(Vdot)
  ventilation_zone 10/1("[S]") -> "[S10]"/1
  Constant 6/1 -> ventilation_zone 10/Enable
  Constant 8/1 -> Product/1
  Product/1 -> ventilation_zone 7/3(Vdot)
  Constant 17/1 -> Product/2
  Constant 5/1 -> Product1/1
  Constant 20/1 -> Product1/2
  Constant 9/1 -> Product2/1
  Constant 23/1 -> Product2/2
  Constant 12/1 -> Product3/1
  Constant 26/1 -> Product3/2
  AIB6/1 -> ventilation_zone 6/1(AIB)
  ventilation_zone 6/1("[S]") -> "[S6]"/1
  Constant 13/1 -> ventilation_zone 6/Enable
  Constant 15/1 -> Product4/1
  Product4/1 -> ventilation_zone 6/3(Vdot)
  Constant 14/1 -> Product4/2
  AIB5/1 -> ventilation_zone 5/1(AIB)
  ventilation_zone 5/1("[S]") -> "[S5]"/1
  Constant 16/1 -> ventilation_zone 5/Enable
  Constant 18/1 -> Product5/1
  Product5/1 -> ventilation_zone 5/3(Vdot)
  Constant 10/1 -> Product5/2
  AIB4/1 -> ventilation_zone 4/1(AIB)
  ventilation_zone 4/1("[S]") -> "[S4]"/1
  Constant 19/1 -> ventilation_zone 4/Enable
  Constant 21/1 -> Product6/1
  Product6/1 -> ventilation_zone 4/3(Vdot)
  Constant 7/1 -> Product6/2
  AIB3/1 -> ventilation_zone 3/1(AIB)
  ventilation_zone 3/1("[S]") -> "[S3]"/1
  Constant 22/1 -> ventilation_zone 3/Enable
  Constant 24/1 -> Product7/1
  Product7/1 -> ventilation_zone 3/3(Vdot)
  Constant 4/1 -> Product7/2
  AIB2/1 -> ventilation_zone 2/1(AIB)
  ventilation_zone 2/1("[S]") -> "[S2]"/1
  Constant 25/1 -> ventilation_zone 2/Enable
  Constant 27/1 -> Product8/1
  Product8/1 -> ventilation_zone 2/3(Vdot)
  Constant 2/1 -> Product8/2
  AIB1/1 -> ventilation_zone 1/1(AIB)
  ventilation_zone 1/1("[S]") -> "[S1]"/1
  Constant 28/1 -> ventilation_zone 1/Enable
  WDB/1 -> ventilation_zone 1/2(WDB), ventilation_zone 2/2(WDB), ventilation_zone 3/2(WDB), ventilation_zone 4/2(WDB), ventilation_zone 5/2(WDB), ventilation_zone 6/2(WDB), ventilation_zone 7/2(WDB), ventilation_zone 8/2(WDB), ventilation_zone 10/2(WDB), ventilation_zone 9/2(WDB)
  Constant 30/1 -> Product9/1
  Product9/1 -> ventilation_zone 1/3(Vdot)
  Constant 29/1 -> Product9/2
  Bus Creator/1 -> "[HVACbus]"/1  "HVAC_2001"
  ventilation_zone 1/2("[HVAC]") -> Bus Creator/1  "z1"
  ventilation_zone 2/2("[HVAC]") -> Bus Creator/2  "z2"
  ventilation_zone 3/2("[HVAC]") -> Bus Creator/3  "z3"
  ventilation_zone 4/2("[HVAC]") -> Bus Creator/4  "z4"
  ventilation_zone 5/2("[HVAC]") -> Bus Creator/5  "z5"
  ventilation_zone 6/2("[HVAC]") -> Bus Creator/6  "z6"
  ventilation_zone 7/2("[HVAC]") -> Bus Creator/7  "z7"
  ventilation_zone 8/2("[HVAC]") -> Bus Creator/8  "z8"
  ventilation_zone 9/2("[HVAC]") -> Bus Creator/9  "z9"
  ventilation_zone 10/2("[HVAC]") -> Bus Creator/10  "z10"

== system carnotUIBK/HVAC/HVAC_9001_window shading ==
  WDB : Inport
  Bus Selector : BusSelector  OutputSignals=Solar_Radiation_beam_normal
  Switch : Switch  Criteria=u2 > Threshold  Threshold=hvac.window(1).I_glob
  Switch1 : Switch  Criteria=u2 > Threshold  Threshold=hvac.window(2).I_glob
  Switch2 : Switch  Criteria=u2 > Threshold  Threshold=hvac.window(3).I_glob
  Switch3 : Switch  Criteria=u2 > Threshold  Threshold=hvac.window(4).I_glob
  Switch4 : Switch  Criteria=u2 > Threshold  Threshold=hvac.window(5).I_glob
  Switch5 : Switch  Criteria=u2 > Threshold  Threshold=hvac.window(6).I_glob
  Transfer Fcn (with initial states) : Subsystem  mask(Transfer Function with Initial States){N=[1], D=[600 1], X0=0}
      mask prompts: N "Numerator:"; D "Denominator:"; X0 "Initial conditions:"
      mask help: Vector expressions for numerator, and denominator. Coefficients are in descending powers of s.
      mask init:
      | [A,B,C,Dd]=tf2ss(N,D);if (isempty(X0));[m,n]=size(A);X0=zeros(1,m); end;
      mask Help: Specify the initial states for the transfer function.  The state ordering is determined by the m-file tf2ss.  There is no unique mapping of the states in a transfer function to states in a state-space representation.  However, tf2ss will consistently use the same mapping for a given transfer function.
      mask Display: dpoly(N,D,'s')
  Window shading zone 1 : carnot/Load/General/Repeating_Profile  period=hvac.window(1).timevalues(end)  rep_seq_t=hvac.window(1).timevalues(1:end-1)  rep_seq_d=hvac.window(1).timeduration  rep_seq_y=hvac.window(1).values
  Window shading zone 2 : carnot/Load/General/Repeating_Profile  period=hvac.window(2).timevalues(end)  rep_seq_t=hvac.window(2).timevalues(1:end-1)  rep_seq_d=hvac.window(2).timeduration  rep_seq_y=hvac.window(2).values
  Window shading zone 3 : carnot/Load/General/Repeating_Profile  period=hvac.window(3).timevalues(end)  rep_seq_t=hvac.window(3).timevalues(1:end-1)  rep_seq_d=hvac.window(3).timeduration  rep_seq_y=hvac.window(3).values
  Window shading zone 4 : carnot/Load/General/Repeating_Profile  period=hvac.window(4).timevalues(end)  rep_seq_t=hvac.window(4).timevalues(1:end-1)  rep_seq_d=hvac.window(4).timeduration  rep_seq_y=hvac.window(4).values
  Window shading zone 5 : carnot/Load/General/Repeating_Profile  period=hvac.window(5).timevalues(end)  rep_seq_t=hvac.window(5).timevalues(1:end-1)  rep_seq_d=hvac.window(5).timeduration  rep_seq_y=hvac.window(5).values
  Window shading zone 6 : carnot/Load/General/Repeating_Profile  period=hvac.window(6).timevalues(end)  rep_seq_t=hvac.window(6).timevalues(1:end-1)  rep_seq_d=hvac.window(6).timeduration  rep_seq_y=hvac.window(6).values
  no shading : Constant  Value=0
  ctrl 1 : Outport
  ctrl 2 : Outport  Port=2
  ctrl 3 : Outport  Port=3
  ctrl 4 : Outport  Port=4
  ctrl 5 : Outport  Port=5
  ctrl 6 : Outport  Port=6
  wires:
  WDB/1 -> Bus Selector/1
  Switch/1 -> ctrl 1/1
  Window shading zone 1/1 -> Switch/1
  Bus Selector/1 -> Transfer Fcn (with initial states)/1(In1)  "<Solar_Radiation_beam_normal>"
  Switch3/1 -> ctrl 4/1
  Window shading zone 4/1 -> Switch3/1
  Switch1/1 -> ctrl 2/1
  Window shading zone 2/1 -> Switch1/1
  Switch4/1 -> ctrl 5/1
  Window shading zone 5/1 -> Switch4/1
  Switch5/1 -> ctrl 6/1
  Window shading zone 6/1 -> Switch5/1
  no shading/1 -> Switch5/3, Switch4/3, Switch3/3, Switch2/3, Switch/3, Switch1/3
  Switch2/1 -> ctrl 3/1
  Window shading zone 3/1 -> Switch2/1
  Transfer Fcn (with initial states)/1(Out1) -> Switch2/2, Switch3/2, Switch5/2, Switch4/2, Switch1/2, Switch/2

== system carnotUIBK/HVAC/HVAC_9002_window opening ==
  WDB : Inport
  AIB window 1 : Inport  Port=2
  AIB window 2 : Inport  Port=3
  AIB window 3 : Inport  Port=4
  AIB window 4 : Inport  Port=5
  AIB window 5 : Inport  Port=6
  AIB window 6 : Inport  Port=7
  Constant 1 : Constant  Value=hvac.window(2).setpoint  VectorParams1D=off
  Constant 2 : Constant  Value=hvac.window(3).setpoint  VectorParams1D=off
  Constant 3 : Constant  Value=hvac.window(4).setpoint  VectorParams1D=off
  Constant 4 : Constant  Value=hvac.window(5).setpoint  VectorParams1D=off
  Constant 5 : Constant  Value=hvac.window(6).setpoint  VectorParams1D=off
  Constant 6 : Constant  Value=hvac.window(1).setpoint  VectorParams1D=off
  on{,1..5} (6 alike) : Constant
  window opening 1 : Subsystem
  window opening 2 : Subsystem
  window opening 3 : Subsystem
  window opening 4 : Subsystem
  window opening 5 : Subsystem
  window opening 6 : Subsystem
  ctrl 1 : Outport
  ctrl 2 : Outport  Port=2
  ctrl 3 : Outport  Port=3
  ctrl 4 : Outport  Port=4
  ctrl 5 : Outport  Port=5
  ctrl 6 : Outport  Port=6
  wires:
  AIB window 1/1 -> window opening 1/2(AIB)
  window opening 1/1(state) -> ctrl 1/1
  on2/1 -> window opening 1/Enable
  AIB window 2/1 -> window opening 2/2(AIB)
  window opening 2/1(state) -> ctrl 2/1
  on1/1 -> window opening 2/Enable
  AIB window 4/1 -> window opening 4/2(AIB)
  window opening 4/1(state) -> ctrl 4/1
  on/1 -> window opening 4/Enable
  AIB window 5/1 -> window opening 5/2(AIB)
  window opening 5/1(state) -> ctrl 5/1
  on3/1 -> window opening 5/Enable
  Constant 6/1 -> window opening 1/1(setpoint)
  AIB window 6/1 -> window opening 6/2(AIB)
  window opening 6/1(state) -> ctrl 6/1
  on4/1 -> window opening 6/Enable
  Constant 1/1 -> window opening 2/1(setpoint)
  Constant 3/1 -> window opening 4/1(setpoint)
  Constant 4/1 -> window opening 5/1(setpoint)
  Constant 5/1 -> window opening 6/1(setpoint)
  WDB/1 -> window opening 6/3(WDB), window opening 5/3(WDB), window opening 4/3(WDB), window opening 3/3(WDB), window opening 2/3(WDB), window opening 1/3(WDB)
  AIB window 3/1 -> window opening 3/2(AIB)
  window opening 3/1(state) -> ctrl 3/1
  on5/1 -> window opening 3/Enable
  Constant 2/1 -> window opening 3/1(setpoint)

== system carnotUIBK/HVAC/HVAC_9003_door opening ==
  profile opening door 1 : carnot/Load/General/Repeating_Profile  period=hvac.door(1).timevalues(end)  rep_seq_t=hvac.door(1).timevalues(1:end-1)  rep_seq_d=hvac.door(1).timeduration  rep_seq_y=hvac.door(1).values
  profile opening door 2 : carnot/Load/General/Repeating_Profile  period=hvac.door(2).timevalues(end)  rep_seq_t=hvac.door(2).timevalues(1:end-1)  rep_seq_d=hvac.door(2).timeduration  rep_seq_y=hvac.door(2).values
  profile opening door 3 : carnot/Load/General/Repeating_Profile  period=hvac.door(3).timevalues(end)  rep_seq_t=hvac.door(3).timevalues(1:end-1)  rep_seq_d=hvac.door(3).timeduration  rep_seq_y=hvac.door(3).values
  profile opening door 4 : carnot/Load/General/Repeating_Profile  period=hvac.door(4).timevalues(end)  rep_seq_t=hvac.door(4).timevalues(1:end-1)  rep_seq_d=hvac.door(4).timeduration  rep_seq_y=hvac.door(4).values
  profile opening door 5 : carnot/Load/General/Repeating_Profile  period=hvac.door(5).timevalues(end)  rep_seq_t=hvac.door(5).timevalues(1:end-1)  rep_seq_d=hvac.door(5).timeduration  rep_seq_y=hvac.door(5).values
  profile opening door 6 : carnot/Load/General/Repeating_Profile  period=hvac.door(6).timevalues(end)  rep_seq_t=hvac.door(6).timevalues(1:end-1)  rep_seq_d=hvac.door(6).timeduration  rep_seq_y=hvac.door(6).values
  ctrl 1 : Outport
  ctrl 2 : Outport  Port=2
  ctrl 3 : Outport  Port=3
  ctrl 4 : Outport  Port=4
  ctrl 5 : Outport  Port=5
  ctrl 6 : Outport  Port=6
  wires:
  profile opening door 1/1 -> ctrl 1/1
  profile opening door 2/1 -> ctrl 2/1
  profile opening door 4/1 -> ctrl 4/1
  profile opening door 5/1 -> ctrl 5/1
  profile opening door 6/1 -> ctrl 6/1
  profile opening door 3/1 -> ctrl 3/1

== system carnotUIBK/HVAC/HVAC_999_TEMPLATE ==
  note: PLEASE CHANGE THE THIS TO THE SYSTEM NUMBER!
  note: 1.	Qdotc: convective power [W]
      | 2.	Qdotr: radiative power [W]
      | 3.	Qdot_S: solar gains [W]
      | 4.	mdot_air: mdot air [kg/s]
      | 5.	mdot_H2O: mdot water [kg/s]
      | 6.	mdot_CO2: mdot CO2 [kg/s]
      | 7.	mdot_VOC: mdot VOC [not used]
      | 8.	Qdot_T_opaque: opaque transmission losses [W]
      | 9.	Qdot_T_ground: ground transmission losses [W]
      | 10.	Qdot_T_neighbour: neighbour transmission losses [W]
      | 11.	Qdot_T_window: window transmission losses [W]
      | 12.	Qdot_V_mech: mechanical ventilation losses [W]
      | 13.	Qdot_V_window: window ventilation losses [W]
      | 14.	Qdot_V_infiltration: infiltration ventilation losses [W]
      | 15.	Qdot_I_person: person internal gains [W]
      | 16.	Qdot_I_light: light internal gains [W]
      | 17.	Qdot_I_electricity: electricity internal gains [W]
      | 18.	Qdot_H: heating power [W]
      | 19.	Qdot_C: cooling power [W]
  WDB : Inport
  AIB1 : Inport  Port=2
  AIB2 : Inport  Port=3
  Bus Creator : BusCreator  Inputs=2
  Bus Selector1 : BusSelector  OutputSignals=Temperature_Ambient
  Bus Selector3 : BusSelector  OutputSignals=Ts
  Integrator : Integrator
  Mux3 : Mux  Inputs=[1 1 15 1 1]
  PID controller : simulink/Continuous/PID Controller  Controller=PI  Form=Ideal  TimeDomain=Continuous-time  SampleTime=-1  IntegratorMethod=Forward Euler  FilterMethod=Forward Euler  ControllerParametersSource=internal  P=hvac.PID.Kp  I=(1/(hvac.PID.Tn*60))  D=0  UseFilter=on  N=100  TunerSelectOption=Transfer Function Based (PID Tuner App)  InitialConditionSource=internal  InitialConditionForIntegrator=0  InitialConditionForFilter=0  DifferentiatorICPrevScaledInput=0  ExternalReset=none  TrackingMode=off  Kt=1  LimitOutput=on  UpperSaturationLimit=hvac.valves.valve_up  LowerSaturationLimit=hvac.valves.valve_low  LinearizeAsGain=off  AntiWindupMode=clamping  Kb=1  POutMin=[]  POutMax=[]  IOutMin=[]  IOutMax=[]  DOutMin=[]  DOutMax=[]  NOutMin=[]  NOutMax=[]  SumOutMin=[]  SumOutMax=[]  SaturationOutMin=[]  SaturationOutMax=[]  PParamMin=[]  PParamMax=[]  IParamMin=[]  IParamMax=[]  DParamMin=[]  DParamMax=[]  NParamMin=[]  NParamMax=[]  KbParamMin=[]  KbParamMax=[]  KtParamMin=[]  KtParamMax=[]  KbOutMin=[]  KbOutMax=[]  KtOutMin=[]  KtOutMax=[]  IntegratorOutMin=[]  IntegratorOutMax=[]  FilterOutMin=[]  FilterOutMax=[]  SumI1OutMin=[]  SumI1OutMax=[]  SumI2OutMin=[]  SumI2OutMax=[]  SumI3OutMin=[]  SumI3OutMax=[]  SumI4OutMin=[]  SumI4OutMax=[]  SumDOutMin=[]  SumDOutMax=[]  DifferentiatorOutMin=[]  DifferentiatorOutMax=[]  FilterDiffOutCoefMin=[]  FilterDiffOutCoefMax=[]  ReciprocalOutMin=[]  ReciprocalOutMax=[]  SumDenOutMin=[]  SumDenOutMax=[]  SumNumOutMin=[]  SumNumOutMax=[]  DivideOutMin=[]  DivideOutMax=[]  IntegratorContinuousStateAttributes=''  IntegratorStateMustResolveToSignalObject=off  IntegratorRTWStateStorageClass=Auto  FilterContinuousStateAttributes=''  FilterStateMustResolveToSignalObject=off  FilterRTWStateStorageClass=Auto  ParallelPVariant=Passthrough  IdealPVariant=InternalParameters  IVariant=InternalParameters  DVariant=Disabled  IntegratorVariant=Continuous  SatVariant=Enabled  AWVariant=ContClampingIdeal  PCopyVariant=InternalParamsIdeal  TRVariant=Disabled  FdbkBlocksVariant=Forward  IdealPFdbkVariant=Disabled  SatFdbkVariant=Disabled  DerivativeFilterVariant=Disabled  NVariant=Disabled  NCopyVariant=Disabled_SignalSpec  FilterICVariant=Disabled  IntegratorICVariant=InternalICs  ExternalResetVariant=Disabled  TRSumVariant=Passthrough  SumFdbkVariant=Disabled  SumVariant=Sum_PI
  Product4 : Product
  Sum1 : Sum  Inputs=|+-
  Terminator : Terminator
  Terminator1 : Terminator
  Transfer Fcn (with initial states)1 : Subsystem  mask(Transfer Function with Initial States){N=[1], D=[300  1], X0=0}
      mask prompts: N "Numerator:"; D "Denominator:"; X0 "Initial conditions:"
      mask help: Vector expressions for numerator, and denominator. Coefficients are in descending powers of s.
      mask init:
      | [A,B,C,Dd]=tf2ss(N,D);if (isempty(X0));[m,n]=size(A);X0=zeros(1,m); end;
      mask Help: Specify the initial states for the transfer function.  The state ordering is determined by the m-file tf2ss.  There is no unique mapping of the states in a transfer function to states in a state-space representation.  However, tf2ss will consistently use the same mapping for a given transfer function.
      mask Display: dpoly(N,D,'s')
  convective : Gain  Gain=0.5  SaturateOnIntegerOverflow=on  OutDataTypeStr=Inherit: Same as input  ParamDataTypeStr=Inherit: Same as input
  heatload : Constant  Value=hvac.heatload
  radiative : Gain  Gain=0.5  SaturateOnIntegerOverflow=on  OutDataTypeStr=Inherit: Same as input  ParamDataTypeStr=Inherit: Same as input
  set point : Constant  Value=hvac.setpoint  VectorParams1D=off
  zeros : Constant  Value=zeros(1,15)
  zeros1 : Constant  Value=zeros(1,1)
  zeros2 : Constant  Value=zeros(1,19)
  "[S1]" : Outport  InitialOutput=0
  "[S2]" : Outport  Port=2  InitialOutput=0
  "[HVACbus]" : Outport  Port=3  InitialOutput=0
  wires:
  Product4/1 -> radiative/1, convective/1, Mux3/4, Bus Creator/1, Integrator/1  "heating power"
  zeros/1 -> Mux3/3
  radiative/1 -> Mux3/1
  convective/1 -> Mux3/2
  heatload/1 -> Product4/2
  PID controller/1 -> Transfer Fcn (with initial states)1/1(In1)
  Bus Selector3/1 -> Sum1/1  "<Ts>"
  set point/1 -> Sum1/2
  Sum1/1 -> PID controller/1
  Mux3/1 -> "[S1]"/1
  WDB/1 -> Bus Selector1/1
  Transfer Fcn (with initial states)1/1(Out1) -> Product4/1
  zeros1/1 -> Mux3/5
  AIB1/1 -> Bus Selector3/1
  Bus Selector1/1 -> Terminator/1  "<Temperature_Ambient>"
  zeros2/1 -> "[S2]"/1
  AIB2/1 -> Terminator1/1
  Bus Creator/1 -> "[HVACbus]"/1  "HVAC_999"
  Integrator/1 -> Bus Creator/2  "heating energy"

== system carnotUIBK/airexchange_intersection/EMPTY ==
  AIB1 : Inport
  AIB2 : Inport  Port=2
  control : Inport  Port=3
  Constant{,1..12,17..19} (16 alike) : Constant  Value=0
  Constant13 : Constant  Value=zeros(1,6)
  Constant14 : Constant  Value=zeros(1,5)
  Constant15 : Constant  Value=zeros(1,6)
  Constant16 : Constant  Value=zeros(1,5)
  Mux1 : Mux  Inputs=[1 1 1 1 1 1 1 6 1 5]
  Mux2 : Mux  Inputs=[1 1 1 1 1 1 1 6 1 5]
  Selector1 : Selector  InputPortWidth=NUMBEROFCONTROLS  IndexOptions=Index vector (dialog)  Indices=[control]  OutputSizes=1
  Terminator : Terminator
  Terminator1 : Terminator
  Terminator2 : Terminator
  "[S1]" : Outport  InitialOutput=0
  "[S2]" : Outport  Port=2  InitialOutput=0
  wires:
  Constant1/1 -> Mux1/4
  Constant4/1 -> Mux1/9
  Constant3/1 -> Mux1/6
  Constant2/1 -> Mux1/5
  Constant/1 -> Mux1/1
  Mux1/1 -> "[S1]"/1
  AIB2/1 -> Terminator2/1
  AIB1/1 -> Terminator1/1
  Constant11/1 -> Mux1/3
  Constant10/1 -> Mux1/2
  Constant12/1 -> Mux1/7
  Constant13/1 -> Mux1/8
  Constant14/1 -> Mux1/10
  control/1 -> Selector1/1
  Selector1/1 -> Terminator/1
  Mux2/1 -> "[S2]"/1
  Constant6/1 -> Mux2/4
  Constant19/1 -> Mux2/9
  Constant18/1 -> Mux2/6
  Constant17/1 -> Mux2/5
  Constant5/1 -> Mux2/1
  Constant8/1 -> Mux2/3
  Constant7/1 -> Mux2/2
  Constant9/1 -> Mux2/7
  Constant15/1 -> Mux2/8
  Constant16/1 -> Mux2/10
